simulink model "SImScape_Bipolarhvdc_Par2"  (R2024b)
settings: Solver=FixedStepDiscrete  StartTime=0.0  StopTime=6  FixedStep=Ts  RelTol=1e-3  AbsTol=1e-2
PostLoadFcn:
  | Ts=50e-6;Tctrl=1*Ts;Rsnu=100;Csnu=2e-6;dec=1;lim=50000;RonInv=0.01; RoffInv=1e5;VfInv=20;
InitFcn:
  | Ts=50e-6;Tctrl=1*Ts;Rsnu=100;Csnu=2e-6;dec=1;lim=50000;RonInv=0.01; RoffInv=1e5;VfInv=20;
libraries: simetranss x1
Description:
  | The 'Model  initialization function' defined in the
  | 
  | Model Properties automatically sets the sample time
  | 
  | Ts to 50e-6 s
settings Model: ARTEMISmethode_block_infos=$$__separator__$$  ModifiedByFormat=Kyle  ExplicitPartitioning=on  Creator=Kyle  LastModifiedBy=Kyle
settings SolverCC: AutoScaleAbsTol=off  ConcurrentTasks=on  AlgebraicLoopSolver=TrustRegion
settings DataIOCC: SaveFormat=Array  SignalLoggingSaveFormat=ModelDataLogs  SaveOutput=off  SignalLogging=off  DSMLogging=off  SaveTime=off  ReturnWorkspaceOutputs=off  SignalLoggingName=sigsOut
settings OptimizationCC: BlockReduction=off  BooleanDataType=off  OptimizeBlockIOStorage=off  BufferReuse=off  GlobalBufferReuse=off  ExpressionFolding=off  ExpressionDepthLimit=2147483647  LocalBlockOutputs=off  InitFltsAndDblsToZero=on  LifeSpan=inf
settings DebuggingCC: SaveWithParameterizedLinksMsg=none  UnderspecifiedInitializationDetection=Classic  MergeDetectMultiDrivingBlocksExec=none  CheckExecutionContextPreStartOutputMsg=on  SignalResolutionControl=TryResolveAllWithWarning  FcnCallInpInsideContextMsg=warning  UnconnectedLineMsg=warning  AllowSymbolicDim=off  StateNameClashWarn=warning  SFUnexpectedBacktrackingDiag=warning  SFNoUnconditionalDefaultTransitionDiag=warning  SFExecutionAtInitializationDiag=none  ArithmeticOperatorsInVariantConditions=warning
settings HardwareCC: ProdBitPerPointer=32  ProdBitPerSizeT=32  ProdBitPerPtrDiffT=32  ProdLargestAtomicFloat=None  ProdIntDivRoundTo=Undefined  ProdEndianess=Unspecified  ProdWordSize=32  ProdHWDeviceType=32-bit Generic  TargetHWDeviceType=32-bit Generic  ProdEqTarget=off
settings ModelReferenceCC: EnableRefExpFcnMdlSchedulingChecks=on  PropagateSignalLabelsOutOfModel=off
settings SFSimCC: SimUseLocalCustomCode=off  CustomCodeUndefinedFunction=UseInterfaceOnly
settings RTWCC: RTWUseLocalCustomCode=off  GPUComputeCapability=3.5
settings CodeAppCC: StateflowObjectComments=on
settings GRTTargetCC: TargetFcnLib=ansi_tfl_tmw.mat  TargetLangStandard=C89/C90 (ANSI)  CombineOutputUpdateFcns=off  GRTInterface=on
settings ConfigComp: CovMetricSettings=dw  CovSaveCumulativeToWorkspaceVar=on  CovSaveSingleToWorkspaceVar=on  CovExternalEMLEnable=off
settings SimscapeCC: SimscapeNormalizeSystem=off

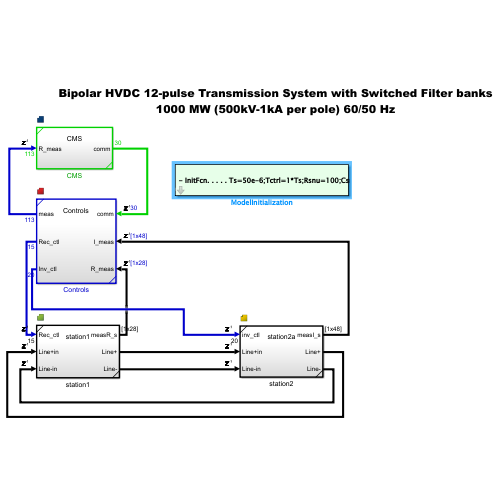
[thumbnail: Simulink's stored preview of the top-level diagram]
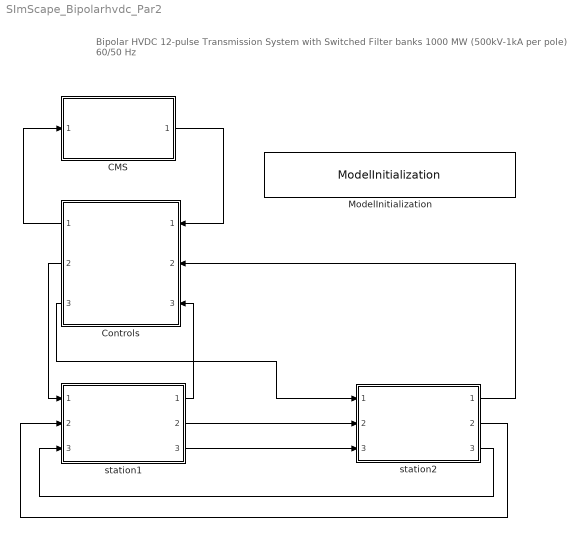
== system SImScape_Bipolarhvdc_Par2 ==
  note: Bipolar HVDC 12-pulse Transmission System with Switched Filter banks
      | 1000 MW (500kV-1kA per pole) 60/50 Hz
  CMS : Subsystem  TreatAsAtomicUnit=on  SystemSampleTime=Ts  ReferencedSubsystem=CMS
  Controls : Subsystem  TreatAsAtomicUnit=on  SystemSampleTime=Ts  ReferencedSubsystem=Controls
  ModelInitialization : simetranss/Usefulls/ModelInitialization  InitFcnX=Ts=50e-6;Tctrl=1*Ts;Rsnu=100;Csnu=2e-6;dec=1;lim=50000;RonInv=0.01; RoffInv=1e5;VfInv=20;  prel=off  posl=on  inif=on  strf=off
  station1 : Subsystem  TreatAsAtomicUnit=on  SystemSampleTime=Ts  ReferencedSubsystem=station1
  station2 : Subsystem  TreatAsAtomicUnit=on  SystemSampleTime=Ts  ReferencedSubsystem=station2a
  wires:
  station1/1 -> Controls/3
  Controls/2 -> station1/1
  Controls/1 -> CMS/1
  CMS/1 -> Controls/1
  Controls/3 -> station2/1
  station2/1 -> Controls/2
  station1/2 -> station2/2
  station1/3 -> station2/3
  station2/2 -> station1/2
  station2/3 -> station1/3
